simulink library "INT_HndBrk_DD"  (R2016b)
settings: Solver=VariableStepAuto  StartTime=0.0  StopTime=10.0  RelTol=1e-3
settings Model: Creator=Administrator  LastModifiedBy=Administrator

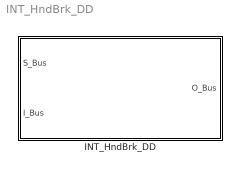
== system INT_HndBrk_DD ==
  INT_HndBrk_DD : Subsystem

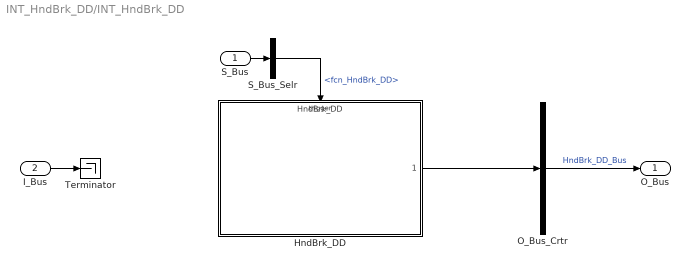
== system INT_HndBrk_DD/INT_HndBrk_DD ==
  S_Bus : Inport
  I_Bus : Inport  Port=2
  HndBrk_DD : ModelReference  ModelNameDialog=HndBrk_DD  SimulationMode=Normal  ModelReferenceVersion=1.2  TriggerPortName=function  TriggerPortTriggerType=function-call  TriggerPortStatesWhenEnabling=held
  O_Bus_Crtr : BusCreator  Inputs=1
  S_Bus_Selr : BusSelector  OutputSignals=fcn_HndBrk_DD
  Terminator : Terminator
  O_Bus : Outport
  wires:
  S_Bus_Selr/1 -> HndBrk_DD/Trigger  "<fcn_HndBrk_DD>"
  S_Bus/1 -> S_Bus_Selr/1
  I_Bus/1 -> Terminator/1
  O_Bus_Crtr/1 -> O_Bus/1  "HndBrk_DD_Bus"
  HndBrk_DD/1 -> O_Bus_Crtr/1
